simulink model "Md28StEnCtrl"  (R2024b)
settings: Solver=FixedStepDiscrete  StartTime=0.0  StopTime=10.0  FixedStep=0.01  RelTol=1e-3
undefined symbols (not defined in the file or in its folder): data, SecRwRtStBkReclnEn_Clear, SecRwRtStBkReclnEn_Set, ThdRwRtStBkReclnEn_Clear, ThdRwRtStBkReclnEn_Set, ThdRwRtStCshnFldEn_Clear, ThdRwRtStCshnFldEn_Set, ThdRwRtStFwdBkwdEn_Clear, ThdRwRtStFwdBkwdEn_Set
libraries: simulink x1
settings Model: Creator=sn55gm  LastModifiedBy=sn55gm
settings SolverCC: AlgebraicLoopSolver=TrustRegion
settings DataIOCC: SaveFormat=StructureWithTime  ReturnWorkspaceOutputs=off
settings OptimizationCC: DefaultParameterBehavior=Inlined  EnhancedBackFolding=on  PassReuseOutputArgsAs=Individual arguments  ZeroExternalMemoryAtStartup=off  ZeroInternalMemoryAtStartup=off  OptimizeBlockOrder=speed  DifferentSizesBufferReuse=on  OptimizationCustomize=off  EfficientTunableParamExpr=on
settings DebuggingCC: ParameterTunabilityLossMsg=error  UnconnectedInputMsg=warning  UnconnectedOutputMsg=warning  UnconnectedLineMsg=warning  ArithmeticOperatorsInVariantConditions=warning
settings ModelReferenceCC: EnableRefExpFcnMdlSchedulingChecks=on  ModelReferenceNumInstancesAllowed=Single
settings SFSimCC: MATLABDynamicMemAlloc=off  CustomCodeUndefinedFunction=UseInterfaceOnly
settings RTWCC: Description=AUTOSAR  SystemTargetFile=autosar.tlc  GenCodeOnly=on  TemplateMakefile=ert_default_tmf  GenerateReport=on  IncludeHyperlinkInReport=on  LaunchReport=on  DataTypeReplacement=CDataTypesFixedWidth  GenerateTraceInfo=on  GenerateTraceReport=on  GenerateTraceReportSl=on  GenerateTraceReportSf=on  GenerateTraceReportEml=on  GPUComputeCapability=3.5
settings CodeAppCC: ForceParamTrailComments=on  IgnoreCustomStorageClasses=off  OperatorAnnotations=on  SimulinkDataObjDesc=on  SFDataObjDesc=on  InsertBlockDesc=on
settings STFCustomTargetCC: TargetLangStandard=C99 (ISO)  MultiwordLength=256  ParMdlRefBuildCompliant=on  CompOptLevelCompliant=on  IncludeMdlTerminateFcn=off  CombineOutputUpdateFcns=on  SuppressErrorStatus=on  ERTCustomFileBanners=on  SupportNonFinite=off  SupportComplex=off  SupportContinuousTime=off  SupportNonInlinedSFcns=off  RemoveResetFunc=on  MATLABClassNameForMDSCustomization=Simulink.SoftwareTarget.ERTCustomization  AutosarCompliant=on  UseToolchainInfoCompliant=on  LookupTableObjectStructAxisOrder=2,1,3,4,...  LUTObjectStructOrderEvenSpacing=Size,Table,Breakpoints  SystemTargetFile=autosar.tlc
settings ERTTargetCC: TargetLangStandard=C99 (ISO)  ConcurrentExecutionCompliant=off  IncludeMdlTerminateFcn=off  SuppressErrorStatus=on  SupportNonFinite=off  SupportComplex=off  ModelStepFunctionPrototypeControlCompliant=off  CPPClassGenCompliant=off  AutosarCompliant=on  LookupTableObjectStructAxisOrder=2,1,3,4,...  LUTObjectStructOrderEvenSpacing=Size,Table,Breakpoints  ERTCustomFileTemplate=example_file_process.tlc  ERTFilePackagingFormat=Compact  BooleanTrueId=TRUE  BooleanFalseId=FALSE  DynamicArrayContainerType=coder::array

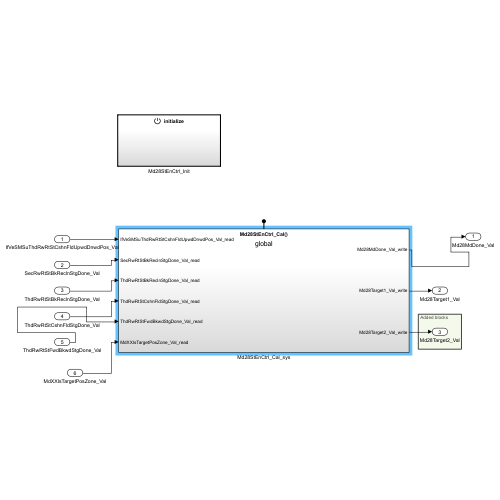
[thumbnail: Simulink's stored preview of the top-level diagram]
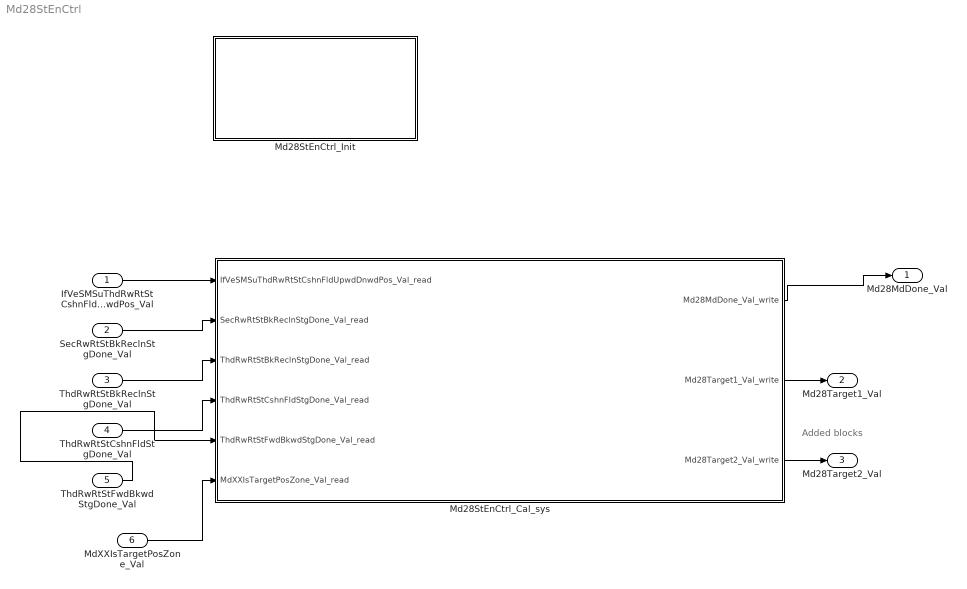
== system Md28StEnCtrl ==
  note: Added blocks
  IfVeSMSuThdRwRtStCshnFldUpwdDnwdPos_Val : Inport  OutDataTypeStr=uint16  PortDimensions=1
  SecRwRtStBkReclnStgDone_Val : Inport  Port=2  OutDataTypeStr=boolean  PortDimensions=1
  ThdRwRtStBkReclnStgDone_Val : Inport  Port=3  OutDataTypeStr=boolean  PortDimensions=1
  ThdRwRtStCshnFldStgDone_Val : Inport  Port=4  OutDataTypeStr=boolean  PortDimensions=1
  ThdRwRtStFwdBkwdStgDone_Val : Inport  Port=5  OutDataTypeStr=boolean  PortDimensions=1
  MdXXIsTargetPosZone_Val : Inport  Port=6  OutDataTypeStr=uint32  PortDimensions=1
  Md28StEnCtrl_Cal_sys : Subsystem
  Md28StEnCtrl_Init : Subsystem
  Md28MdDone_Val : Outport  OutDataTypeStr=uint8  PortDimensions=1  VectorParamsAs1DForOutWhenUnconnected=off
  Md28Target1_Val : Outport  Port=2  OutDataTypeStr=boolean  PortDimensions=1  VectorParamsAs1DForOutWhenUnconnected=off
  Md28Target2_Val : Outport  Port=3  OutDataTypeStr=boolean  PortDimensions=1  VectorParamsAs1DForOutWhenUnconnected=off
  wires:
  IfVeSMSuThdRwRtStCshnFldUpwdDnwdPos_Val/1 -> Md28StEnCtrl_Cal_sys/1(IfVeSMSuThdRwRtStCshnFldUpwdDnwdPos_Val_read)
  SecRwRtStBkReclnStgDone_Val/1 -> Md28StEnCtrl_Cal_sys/2(SecRwRtStBkReclnStgDone_Val_read)
  ThdRwRtStBkReclnStgDone_Val/1 -> Md28StEnCtrl_Cal_sys/3(ThdRwRtStBkReclnStgDone_Val_read)
  ThdRwRtStCshnFldStgDone_Val/1 -> Md28StEnCtrl_Cal_sys/4(ThdRwRtStCshnFldStgDone_Val_read)
  ThdRwRtStFwdBkwdStgDone_Val/1 -> Md28StEnCtrl_Cal_sys/5(ThdRwRtStFwdBkwdStgDone_Val_read)
  Md28StEnCtrl_Cal_sys/1(Md28MdDone_Val_write) -> Md28MdDone_Val/1
  MdXXIsTargetPosZone_Val/1 -> Md28StEnCtrl_Cal_sys/6(MdXXIsTargetPosZone_Val_read)
  Md28StEnCtrl_Cal_sys/2(Md28Target1_Val_write) -> Md28Target1_Val/1
  Md28StEnCtrl_Cal_sys/3(Md28Target2_Val_write) -> Md28Target2_Val/1

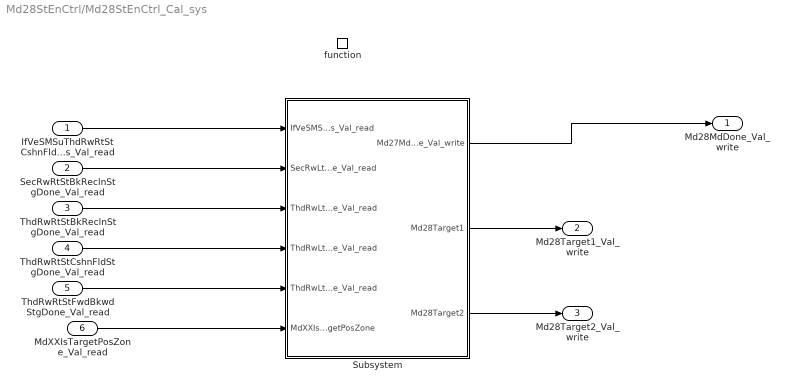
== system Md28StEnCtrl/Md28StEnCtrl_Cal_sys ==
  IfVeSMSuThdRwRtStCshnFldUpwdDnwdPos_Val_read : Inport
  SecRwRtStBkReclnStgDone_Val_read : Inport  Port=2
  ThdRwRtStBkReclnStgDone_Val_read : Inport  Port=3
  ThdRwRtStCshnFldStgDone_Val_read : Inport  Port=4
  ThdRwRtStFwdBkwdStgDone_Val_read : Inport  Port=5
  MdXXIsTargetPosZone_Val_read : Inport  Port=6
  function : TriggerPort  TriggerType=function-call  IsSimulinkFunction=on  FunctionName=Md28StEnCtrl_Cal  VariantControl=(inherit)
  Subsystem : Subsystem
  Md28MdDone_Val_write : Outport  VectorParamsAs1DForOutWhenUnconnected=off
      settings: EnsureOutportIsVirtual=on
  Md28Target1_Val_write : Outport  Port=2  VectorParamsAs1DForOutWhenUnconnected=off
      settings: EnsureOutportIsVirtual=on
  Md28Target2_Val_write : Outport  Port=3  VectorParamsAs1DForOutWhenUnconnected=off
      settings: EnsureOutportIsVirtual=on
  wires:
  IfVeSMSuThdRwRtStCshnFldUpwdDnwdPos_Val_read/1 -> Subsystem/1(IfVeSMSuThdRwLtStCshnFldUpwdDnwdPos_Val_read)
  SecRwRtStBkReclnStgDone_Val_read/1 -> Subsystem/2(SecRwLtStBkReclnStgDone_Val_read)
  ThdRwRtStBkReclnStgDone_Val_read/1 -> Subsystem/3(ThdRwLtStBkReclnStgDone_Val_read)
  ThdRwRtStCshnFldStgDone_Val_read/1 -> Subsystem/4(ThdRwLtStCshnFldStgDone_Val_read)
  ThdRwRtStFwdBkwdStgDone_Val_read/1 -> Subsystem/5(ThdRwLtStFwdBkwdStgDone_Val_read)
  Subsystem/1(Md27MdDone_Val_write) -> Md28MdDone_Val_write/1
  MdXXIsTargetPosZone_Val_read/1 -> Subsystem/6(MdXXIsTargetPosZone)
  Subsystem/2(Md28Target1) -> Md28Target1_Val_write/1
  Subsystem/3(Md28Target2) -> Md28Target2_Val_write/1

== system Md28StEnCtrl/Md28StEnCtrl_Init ==
  Event Listener : EventListener  EventName=reset

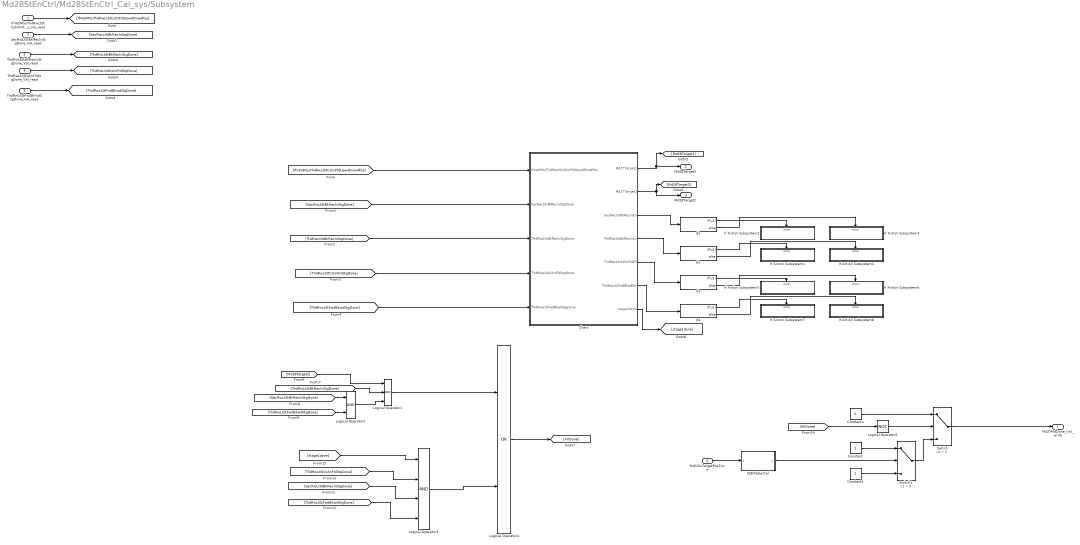
== system Md28StEnCtrl/Md28StEnCtrl_Cal_sys/Subsystem ==
  IfVeSMSuThdRwLtStCshnFldUpwdDnwdPos_Val_read : Inport
  SecRwLtStBkReclnStgDone_Val_read : Inport  Port=2
  ThdRwLtStBkReclnStgDone_Val_read : Inport  Port=3
  ThdRwLtStCshnFldStgDone_Val_read : Inport  Port=4
  ThdRwLtStFwdBkwdStgDone_Val_read : Inport  Port=5
  MdXXIsTargetPosZone : Inport  Port=6
  32BitSelector : Subsystem  mask(32 Bit Selector){BitNum=14}
      mask prompts: BitNum "Select Bit Number"
      mask help: Allows selection of a particular bit (0-31) out of a packed word up to 32 bits long. Output will be true if the bit number selected via the mask parameter is equal to one.
      mask TypeOptions BitNum: 0 | 1 | 2 | 3 | 4 | 5 | 6 | 7 | 8 | 9 | 10 | 11 | 12 | 13 | 14 | 15 | 16 | 17 | 18 | 19 | 20 | 21 | 22 | 23 | 24 | 25 | 26 | 27 | 28 | 29 | 30 | 31
      mask Display:
      | text(0.5, 0.8,'BIT','horizontalAlignment','center')
      | text(0.5, 0.5,'SELECTOR','horizontalAlignment','center')
      | text(0.5, 0.2,['-- Bit ',char(get_param(gcb,'BitNum')),' --'],'horizontalAlignment','center')
  Chart : Stateflow chart  TreatAsAtomicUnit=on
  Constant : Constant  OutDataTypeStr=uint8
  Constant1 : Constant  Value=2  OutDataTypeStr=uint8
  Constant2 : Constant  Value=0  OutDataTypeStr=uint8
  If Action Subsystem1 : Subsystem  TreatAsAtomicUnit=on
  If Action Subsystem2 : Subsystem  TreatAsAtomicUnit=on
  If Action Subsystem3 : Subsystem  TreatAsAtomicUnit=on
  If Action Subsystem4 : Subsystem  TreatAsAtomicUnit=on
  If Action Subsystem5 : Subsystem  TreatAsAtomicUnit=on
  If Action Subsystem6 : Subsystem  TreatAsAtomicUnit=on
  If Action Subsystem7 : Subsystem  TreatAsAtomicUnit=on
  If Action Subsystem8 : Subsystem  TreatAsAtomicUnit=on
  If{1..4} (4 alike) : If  IfExpression=u1
  Logical Operator1 : Logic  Inputs=3  AllPortsSameDT=off  OutDataTypeStr=boolean
  Logical Operator2 : Logic  AllPortsSameDT=off  OutDataTypeStr=boolean
  Logical Operator3 : Logic  Inputs=4  AllPortsSameDT=off  OutDataTypeStr=boolean
  Logical Operator4 : Logic  Operator=OR  AllPortsSameDT=off  OutDataTypeStr=boolean
  Logical Operator5 : Logic  Operator=NOT  AllPortsSameDT=off  OutDataTypeStr=boolean
  Switch : Switch  Criteria=u2 > Threshold  SaturateOnIntegerOverflow=off  InputSameDT=off
  Switch1 : Switch  Criteria=u2 > Threshold  SaturateOnIntegerOverflow=off  InputSameDT=off
  Md27MdDone_Val_write : Outport  VectorParamsAs1DForOutWhenUnconnected=off
      settings: EnsureOutportIsVirtual=on
  Md28Target1 : Outport  Port=2  VectorParamsAs1DForOutWhenUnconnected=off
  Md28Target2 : Outport  Port=3  VectorParamsAs1DForOutWhenUnconnected=off
  wires:
  IfVeSMSuThdRwLtStCshnFldUpwdDnwdPos_Val_read/1 -> [IfVeSMSuThdRwLtStCshnFldUpwdDnwdPos]
  SecRwLtStBkReclnStgDone_Val_read/1 -> [SecRwLtStBkReclnStgDone]
  ThdRwLtStBkReclnStgDone_Val_read/1 -> [ThdRwLtStBkReclnStgDone]
  ThdRwLtStCshnFldStgDone_Val_read/1 -> [ThdRwLtStCshnFldStgDone]
  ThdRwLtStFwdBkwdStgDone_Val_read/1 -> [ThdRwLtStFwdBkwdStgDone]
  [IfVeSMSuThdRwLtStCshnFldUpwdDnwdPos] -> Chart/1(IfVeSMSuThdRwLtStCshnFldUpwdDnwdPos)
  [SecRwLtStBkReclnStgDone] -> Chart/2(SecRwLtStBkReclnStgDone)
  [ThdRwLtStBkReclnStgDone] -> Chart/3(ThdRwLtStBkReclnStgDone)
  [ThdRwLtStCshnFldStgDone] -> Chart/4(ThdRwLtStCshnFldStgDone)
  [ThdRwLtStFwdBkwdStgDone] -> Chart/5(ThdRwLtStFwdBkwdStgDone)
  Chart/1(Md27Target1) -> [Md28Target1], Md28Target1/1
  Chart/2(Md27Target2) -> Md28Target2/1, [Md28Target2]
  Chart/3(SecRwLtStBkReclnEn) -> If1/1
  Chart/4(ThdRwLtStBkReclnEn) -> If2/1
  Chart/5(ThdRwLtStCshnFldEn) -> If3/1
  Chart/6(ThdRwLtStFwdBkwdEn) -> If4/1
  If1/1 -> If Action Subsystem2/Action
  If1/2 -> If Action Subsystem3/Action
  If2/1 -> If Action Subsystem1/Action
  If2/2 -> If Action Subsystem4/Action
  If3/1 -> If Action Subsystem5/Action
  If3/2 -> If Action Subsystem6/Action
  If4/1 -> If Action Subsystem7/Action
  If4/2 -> If Action Subsystem8/Action
  [ThdRwLtStBkReclnStgDone] -> Logical Operator1/2
  [SecRwLtStBkReclnStgDone] -> Logical Operator2/1
  [ThdRwLtStFwdBkwdStgDone] -> Logical Operator2/2
  Logical Operator2/1 -> Logical Operator1/3
  [SecRwLtStBkReclnStgDone] -> Logical Operator3/3
  [ThdRwLtStFwdBkwdStgDone] -> Logical Operator3/4
  [ThdRwLtStCshnFldStgDone] -> Logical Operator3/2
  Logical Operator1/1 -> Logical Operator4/1
  Logical Operator3/1 -> Logical Operator4/2
  Logical Operator4/1 -> [AllDone]
  Logical Operator5/1 -> Switch/2
  Constant/1 -> Switch1/1
  32BitSelector/1(y) -> Switch1/2
  Constant1/1 -> Switch1/3
  Switch/1 -> Md27MdDone_Val_write/1
  MdXXIsTargetPosZone/1 -> 32BitSelector/1(x)
  [AllDone] -> Logical Operator5/1
  Constant2/1 -> Switch/1
  Switch1/1 -> Switch/3
  [Md28Target2] -> Logical Operator1/1
  Chart/7(stage1done) -> [stage1done]
  [stage1done] -> Logical Operator3/1

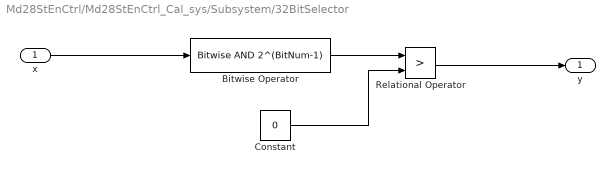
== system Md28StEnCtrl/Md28StEnCtrl_Cal_sys/Subsystem/32BitSelector ==
  x : Inport
  Bitwise Operator : simulink/Logic and Bit Operations/Bitwise Operator  logicop=AND  UseBitMask=on  BitMask=2^(BitNum-1)  BitMaskRealWorld=Stored Integer
  Constant : Constant  Value=0  OutDataTypeStr=uint32
  Relational Operator : RelationalOperator  Operator=>  OutDataTypeStr=boolean  RndMeth=Simplest  InputSameDT=off
  y : Outport  VectorParamsAs1DForOutWhenUnconnected=off
  wires:
  Relational Operator/1 -> y/1
  Constant/1 -> Relational Operator/2
  x/1 -> Bitwise Operator/1
  Bitwise Operator/1 -> Relational Operator/1

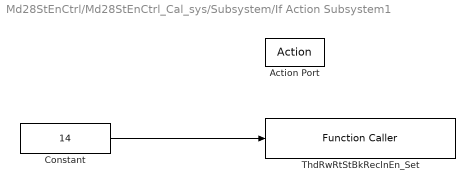
== system Md28StEnCtrl/Md28StEnCtrl_Cal_sys/Subsystem/If Action Subsystem1 ==
  Action Port : ActionPort  ActionPortLabel=if(u1)
  Constant : Constant  Value=14  OutDataTypeStr=uint8
  ThdRwRtStBkReclnEn_Set : FunctionCaller  FunctionPrototype=ThdRwRtStBkReclnEn_Set(data)  InputArgumentSpecifications=uint8(1)  OutputArgumentSpecifications=<Enter example>
  wires:
  Constant/1 -> ThdRwRtStBkReclnEn_Set/1

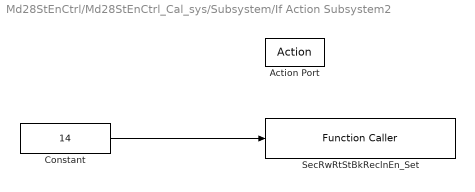
== system Md28StEnCtrl/Md28StEnCtrl_Cal_sys/Subsystem/If Action Subsystem2 ==
  Action Port : ActionPort  ActionPortLabel=if(u1)
  Constant : Constant  Value=14  OutDataTypeStr=uint8
  SecRwRtStBkReclnEn_Set : FunctionCaller  FunctionPrototype=SecRwRtStBkReclnEn_Set(data)  InputArgumentSpecifications=uint8(1)  OutputArgumentSpecifications=<Enter example>
  wires:
  Constant/1 -> SecRwRtStBkReclnEn_Set/1

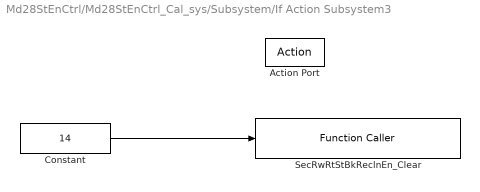
== system Md28StEnCtrl/Md28StEnCtrl_Cal_sys/Subsystem/If Action Subsystem3 ==
  Action Port : ActionPort  ActionPortLabel=else
  Constant : Constant  Value=14  OutDataTypeStr=uint8
  SecRwRtStBkReclnEn_Clear : FunctionCaller  FunctionPrototype=SecRwRtStBkReclnEn_Clear(data)  InputArgumentSpecifications=uint8(1)  OutputArgumentSpecifications=<Enter example>
  wires:
  Constant/1 -> SecRwRtStBkReclnEn_Clear/1

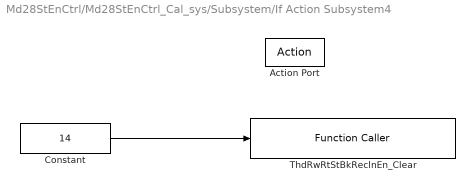
== system Md28StEnCtrl/Md28StEnCtrl_Cal_sys/Subsystem/If Action Subsystem4 ==
  Action Port : ActionPort  ActionPortLabel=else
  Constant : Constant  Value=14  OutDataTypeStr=uint8
  ThdRwRtStBkReclnEn_Clear : FunctionCaller  FunctionPrototype=ThdRwRtStBkReclnEn_Clear(data)  InputArgumentSpecifications=uint8(1)  OutputArgumentSpecifications=<Enter example>
  wires:
  Constant/1 -> ThdRwRtStBkReclnEn_Clear/1

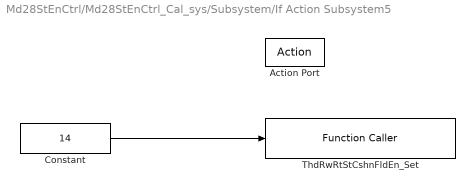
== system Md28StEnCtrl/Md28StEnCtrl_Cal_sys/Subsystem/If Action Subsystem5 ==
  Action Port : ActionPort  ActionPortLabel=if(u1)
  Constant : Constant  Value=14  OutDataTypeStr=uint8
  ThdRwRtStCshnFldEn_Set : FunctionCaller  FunctionPrototype=ThdRwRtStCshnFldEn_Set(data)  InputArgumentSpecifications=uint8(1)  OutputArgumentSpecifications=<Enter example>
  wires:
  Constant/1 -> ThdRwRtStCshnFldEn_Set/1

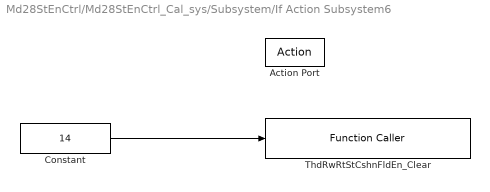
== system Md28StEnCtrl/Md28StEnCtrl_Cal_sys/Subsystem/If Action Subsystem6 ==
  Action Port : ActionPort  ActionPortLabel=else
  Constant : Constant  Value=14  OutDataTypeStr=uint8
  ThdRwRtStCshnFldEn_Clear : FunctionCaller  FunctionPrototype=ThdRwRtStCshnFldEn_Clear(data)  InputArgumentSpecifications=uint8(1)  OutputArgumentSpecifications=<Enter example>
  wires:
  Constant/1 -> ThdRwRtStCshnFldEn_Clear/1

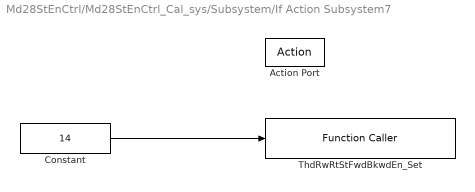
== system Md28StEnCtrl/Md28StEnCtrl_Cal_sys/Subsystem/If Action Subsystem7 ==
  Action Port : ActionPort  ActionPortLabel=if(u1)
  Constant : Constant  Value=14  OutDataTypeStr=uint8
  ThdRwRtStFwdBkwdEn_Set : FunctionCaller  FunctionPrototype=ThdRwRtStFwdBkwdEn_Set(data)  InputArgumentSpecifications=uint8(1)  OutputArgumentSpecifications=<Enter example>
  wires:
  Constant/1 -> ThdRwRtStFwdBkwdEn_Set/1

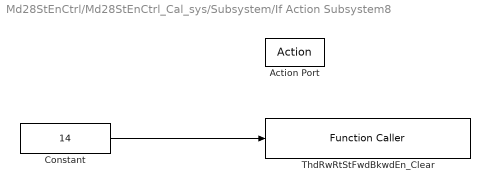
== system Md28StEnCtrl/Md28StEnCtrl_Cal_sys/Subsystem/If Action Subsystem8 ==
  Action Port : ActionPort  ActionPortLabel=else
  Constant : Constant  Value=14  OutDataTypeStr=uint8
  ThdRwRtStFwdBkwdEn_Clear : FunctionCaller  FunctionPrototype=ThdRwRtStFwdBkwdEn_Clear(data)  InputArgumentSpecifications=uint8(1)  OutputArgumentSpecifications=<Enter example>
  wires:
  Constant/1 -> ThdRwRtStFwdBkwdEn_Clear/1

== stateflow chart Md28StEnCtrl/Md28StEnCtrl_Cal_sys/Subsystem/Chart ==
  (default) -> (junction 7) : {SecRwLtStBkReclnEn=0;
      | ThdRwLtStBkReclnEn=0;
      | ThdRwLtStCshnFldEn=0;
      | ThdRwLtStFwdBkwdEn=0;}
  (junction 7) -> (junction 26) [order 1] : [IfVeSMSuThdRwLtStCshnFldUpwdDnwdPos>=4000]
  (junction 7) -> (junction 13) [order 2]
  (junction 26) -> (junction 9) : {Md27Target2=true;}
  (junction 9) -> (junction 16) [order 1] : [~ThdRwLtStBkReclnStgDone]
  (junction 9) -> (junction 18) [order 2]
  (junction 16) -> (junction 20) : {ThdRwLtStBkReclnEn=1;}
  (junction 20) -> (junction 18)
  (junction 18) -> (junction 23)
  (junction 23) -> (junction 25) [order 1] : [~SecRwLtStBkReclnStgDone]
  (junction 23) -> (junction 34) [order 2]
  (junction 25) -> (junction 29) : {SecRwLtStBkReclnEn=1;}
  (junction 34) -> (junction 36) [order 1] : [~ThdRwLtStFwdBkwdStgDone]
  (junction 34) -> (junction 11) [order 2]
  (junction 36) -> (junction 38) : {ThdRwLtStFwdBkwdEn=1;}
  (junction 11) -> (junction 13)
  (junction 38) -> (junction 11)
  (junction 29) -> (junction 38)
  (junction 13) -> (junction 32)
  (junction 32) -> (junction 41) [order 1] : [IfVeSMSuThdRwLtStCshnFldUpwdDnwdPos<4000]
  (junction 32) -> (junction 43) [order 2]
  (junction 41) -> (junction 93) : {Md27Target1=true;}
  (junction 93) -> (junction 94) [order 1] : [~SecRwLtStBkReclnStgDone]
  (junction 93) -> (junction 45) [order 2]
  (junction 94) -> (junction 96) : {SecRwLtStBkReclnEn=1;}
  (junction 45) -> (junction 47) [order 1] : [IfVeSMSuThdRwLtStCshnFldUpwdDnwdPos<4000]
  (junction 45) -> (junction 56) [order 2] : [IfVeSMSuThdRwLtStCshnFldUpwdDnwdPos>=4000]
  (junction 47) -> (junction 51) : {ThdRwLtStCshnFldEn=1;}
  (junction 56) -> (junction 58) [order 1] : [~ThdRwLtStFwdBkwdStgDone]
  (junction 56) -> (junction 60) [order 2]
  (junction 58) -> (junction 59) : {ThdRwLtStFwdBkwdEn=1;}
  (junction 59) -> (junction 60)
  (junction 60) -> (junction 68)
  (junction 68) -> (junction 67) [order 1] : [IfVeSMSuThdRwLtStCshnFldUpwdDnwdPos>=4000]
  (junction 68) -> (junction 72) [order 2]
  (junction 67) -> (junction 71) : {SecRwLtStBkReclnEn=1;
      | stage1done=1;}
  (junction 71) -> (junction 72)
  (junction 72) -> (junction 65)
  (junction 65) -> (junction 78) [order 1] : [~ThdRwLtStBkReclnStgDone]
  (junction 65) -> (junction 52) [order 2]
  (junction 78) -> (junction 79) : {ThdRwLtStBkReclnEn=1;}
  (junction 52) -> (junction 43)
  (junction 79) -> (junction 52)
  (junction 51) -> (junction 79)
  (junction 96) -> (junction 51)
  (junction 43) -> (junction 85)
  data: IfVeSMSuThdRwLtStCshnFldUpwdDnwdPos input; SecRwLtStBkReclnStgDone input; ThdRwLtStBkReclnStgDone input; ThdRwLtStCshnFldStgDone input; ThdRwLtStFwdBkwdStgDone input; Md27Target1 output boolean; Md27Target2 output boolean; SecRwLtStBkReclnEn output; ThdRwLtStBkReclnEn output; ThdRwLtStCshnFldEn output; ThdRwLtStFwdBkwdEn output; stage1done output
